simulink model "Singertank"  (R2020b)
settings: Solver=VariableStepAuto  StartTime=0.0  StopTime=10.0  RelTol=1e-3
settings Model: Creator=ACER  LastModifiedBy=ACER

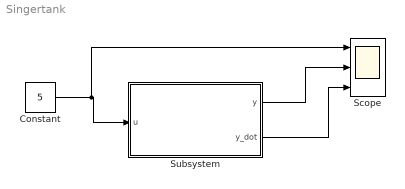
== system Singertank ==
  Constant : Constant  Value=5
  Scope : Scope  NumInputPorts=3
  Subsystem : Subsystem
  wires:
  Constant/1 -> Scope/1, Subsystem/1(u)
  Subsystem/1(y) -> Scope/2
  Subsystem/2(y_dot) -> Scope/3

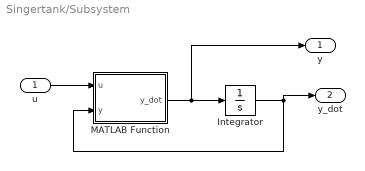
== system Singertank/Subsystem ==
  u : Inport
  Integrator : Integrator
  MATLAB Function : MATLAB Function  TreatAsAtomicUnit=on
  y : Outport
  y_dot : Outport  Port=2
  wires:
  MATLAB Function/1(y_dot) -> y/1, Integrator/1
  Integrator/1 -> MATLAB Function/2(y), y_dot/1
  u/1 -> MATLAB Function/1(u)

== matlab function Singertank/Subsystem/MATLAB Function ==
  data: u input; y_dot output; y input
function y_dot = fcn(u,y)
K=140;
C=0.9;
g=9.81;
A= 314;
y_dot = (K*u -C*sqrt(2*g*y))/A;
